simulink model "costas_loop"  (R2013a)
settings: Solver=ode3  StartTime=0.0  StopTime=10/1200  FixedStep=(1/1200)/1024  RelTol=1e-3
libraries: dsparch4 x3, commsynccomp2 x2, commrandsrc2 x1
settings Model: Creator=tibbs2010  LastModifiedBy=tibbs2010

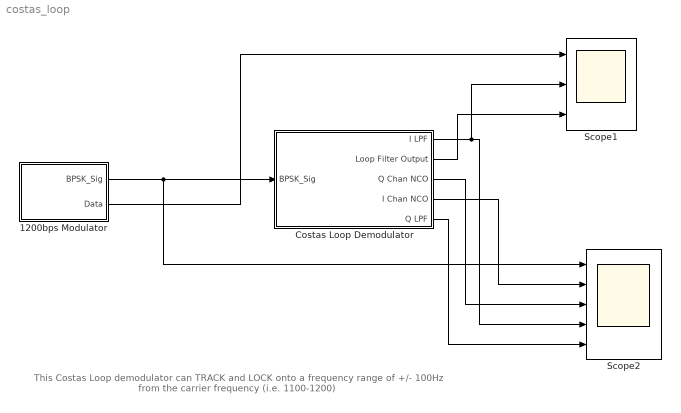
== system costas_loop ==
  note: This Costas Loop demodulator can TRACK and LOCK onto a
      |  frequency range of +/- 100Hz from the carrier frequency (i.e. 1100-1200)
  1200bps Modulator : Subsystem
  Costas Loop Demodulator : Subsystem
  Scope1 : Scope  NumInputPorts=3
      settings: TimeRange=0.5  YMin=-1~-1~-2  YMax=2~1~2
  Scope2 : Scope  NumInputPorts=5
      settings: TimeRange=0.5  YMin=-2~-2~-2~-5~-5  YMax=2~2~2~5~5
  wires:
  1200bps Modulator/1(BPSK_Sig) -> Scope2/1, Costas Loop Demodulator/1(BPSK_Sig)
  1200bps Modulator/2(Data) -> Scope1/1
  Costas Loop Demodulator/1(I LPF) -> Scope1/2, Scope2/4
  Costas Loop Demodulator/2(Loop Filter Output) -> Scope1/3
  Costas Loop Demodulator/4(I Chan NCO) -> Scope2/2
  Costas Loop Demodulator/3(Q Chan NCO) -> Scope2/3
  Costas Loop Demodulator/5(Q LPF) -> Scope2/5

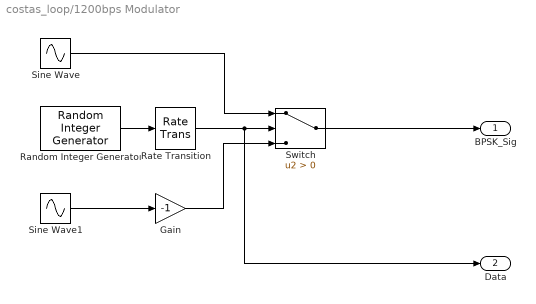
== system costas_loop/1200bps Modulator ==
  Gain : Gain  Gain=-1
  Random Integer Generator : commrandsrc2/Random Integer Generator  mul=2  seed=randseed  Ts=1/1200  frameBased=off  sampPerFrame=1  orient=off  outDataType=double
  Rate Transition : RateTransition
  Sine Wave : Sin  Frequency=2*pi*1200  Phase=pi/2  Samples=1024  SampleTime=(1/1200)/1024
  Sine Wave1 : Sin  Frequency=2*pi*1200  Phase=pi/2  Samples=1024  SampleTime=(1/1200)/1024
  Switch : Switch  Criteria=u2 > Threshold
  BPSK_Sig : Outport
  Data : Outport  Port=2
  wires:
  Switch/1 -> BPSK_Sig/1
  Random Integer Generator/1 -> Rate Transition/1
  Rate Transition/1 -> Data/1, Switch/2
  Sine Wave/1 -> Switch/1
  Sine Wave1/1 -> Gain/1
  Gain/1 -> Switch/3

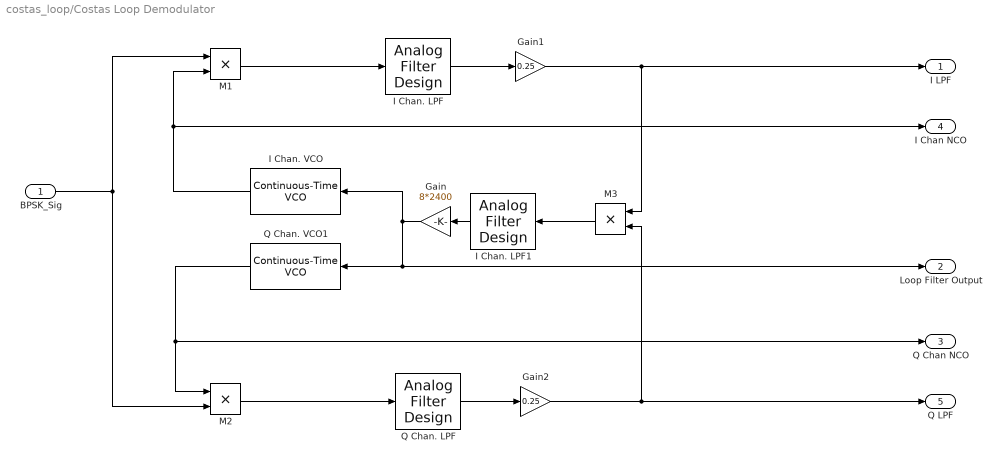
== system costas_loop/Costas Loop Demodulator ==
  BPSK_Sig : Inport
  Gain : Gain  Gain=8*2400
  Gain1 : Gain  Gain=0.25
  Gain2 : Gain  Gain=0.25
  I Chan. LPF : dsparch4/Analog Filter Design  method=Butterworth  filttype=Lowpass  N=1  Wlo=2*pi*2400  Whi=80  Rp=2  Rs=40
  I Chan. LPF1 : dsparch4/Analog Filter Design  method=Butterworth  filttype=Lowpass  N=1  Wlo=2*pi*2400  Whi=80  Rp=2  Rs=40
  I Chan. VCO : commsynccomp2/Continuous-Time VCO  Ac=1  Fc=1100  Kc=1  Ph=0
  M1 : Product
  M2 : Product
  M3 : Product
  Q Chan. LPF : dsparch4/Analog Filter Design  method=Butterworth  filttype=Lowpass  N=1  Wlo=2*pi*2400  Whi=80  Rp=2  Rs=40
  Q Chan. VCO1 : commsynccomp2/Continuous-Time VCO  Ac=1  Fc=1100  Kc=1  Ph=pi/2
  I LPF : Outport
  Loop Filter Output : Outport  Port=2
  Q Chan NCO : Outport  Port=3
  I Chan NCO : Outport  Port=4
  Q LPF : Outport  Port=5
  wires:
  M2/1 -> Q Chan. LPF/1
  M1/1 -> I Chan. LPF/1
  I Chan. LPF/1 -> Gain1/1
  Q Chan. LPF/1 -> Gain2/1
  M3/1 -> I Chan. LPF1/1
  BPSK_Sig/1 -> M1/1, M2/2
  I Chan. VCO/1 -> M1/2, I Chan NCO/1
  Q Chan. VCO1/1 -> M2/1, Q Chan NCO/1
  Gain/1 -> I Chan. VCO/1, Loop Filter Output/1, Q Chan. VCO1/1
  I Chan. LPF1/1 -> Gain/1
  Gain1/1 -> I LPF/1, M3/1
  Gain2/1 -> Q LPF/1, M3/2
